simulink model "test_mdl_NI"  (R2018a)
settings: Solver=VariableStepAuto  StartTime=0.0  StopTime=10.0  RelTol=1e-3
(part 15 of 24)

== system test_mdl_NI/To_NI_HIL/Soft_ABS/WheelSpeed ==
  in : Inport
  WhlFl_W_Meas : Subsystem
  WhlFr_W_Meas : Subsystem
  WhlRl_W_Meas : Subsystem
  WhlRotatFl_No_Cnt : Subsystem
  WhlRotatFr_No_Cnt : Subsystem
  WhlRotatRl_No_Cnt : Subsystem
  WhlRotatRr_No_Cnt : Subsystem
  WhlRr_W_Meas : Subsystem
  bus_creator : BusCreator  Inputs=8
  bus_selector : BusSelector  OutputSignals=WhlFl_W_Meas,WhlFr_W_Meas,WhlRl_W_Meas,WhlRr_W_Meas,WhlRotatFl_No_Cnt,WhlRotatFr_No_Cnt,WhlRotatRl_No_Cnt,WhlRotatRr_No_Cnt
  out_port : Outport
  wires:
  bus_creator/1 -> out_port/1  "WheelSpeed"
  WhlFl_W_Meas/1(out) -> bus_creator/1  "WhlFl_W_Meas"
  WhlFr_W_Meas/1(out) -> bus_creator/2  "WhlFr_W_Meas"
  WhlRl_W_Meas/1(out) -> bus_creator/3  "WhlRl_W_Meas"
  WhlRr_W_Meas/1(out) -> bus_creator/4  "WhlRr_W_Meas"
  WhlRotatFl_No_Cnt/1(out) -> bus_creator/5  "WhlRotatFl_No_Cnt"
  WhlRotatFr_No_Cnt/1(out) -> bus_creator/6  "WhlRotatFr_No_Cnt"
  WhlRotatRl_No_Cnt/1(out) -> bus_creator/7  "WhlRotatRl_No_Cnt"
  WhlRotatRr_No_Cnt/1(out) -> bus_creator/8  "WhlRotatRr_No_Cnt"
  bus_selector/1 -> WhlFl_W_Meas/1(in)  "<WhlFl_W_Meas>"
  bus_selector/2 -> WhlFr_W_Meas/1(in)  "<WhlFr_W_Meas>"
  bus_selector/3 -> WhlRl_W_Meas/1(in)  "<WhlRl_W_Meas>"
  bus_selector/4 -> WhlRr_W_Meas/1(in)  "<WhlRr_W_Meas>"
  bus_selector/5 -> WhlRotatFl_No_Cnt/1(in)  "<WhlRotatFl_No_Cnt>"
  bus_selector/6 -> WhlRotatFr_No_Cnt/1(in)  "<WhlRotatFr_No_Cnt>"
  bus_selector/7 -> WhlRotatRl_No_Cnt/1(in)  "<WhlRotatRl_No_Cnt>"
  bus_selector/8 -> WhlRotatRr_No_Cnt/1(in)  "<WhlRotatRr_No_Cnt>"
  in/1 -> bus_selector/1

== system test_mdl_NI/To_NI_HIL/Soft_ABS/Yaw_Data ==
  in : Inport
  VehYaw_W_Actl : Subsystem
  bus_creator : BusCreator  Inputs=1
  bus_selector : BusSelector  OutputSignals=VehYaw_W_Actl
  out_port : Outport
  wires:
  bus_creator/1 -> out_port/1  "Yaw_Data"
  VehYaw_W_Actl/1(out) -> bus_creator/1  "VehYaw_W_Actl"
  bus_selector/1 -> VehYaw_W_Actl/1(in)  "<VehYaw_W_Actl>"
  in/1 -> bus_selector/1

== system test_mdl_NI/To_NI_HIL/Soft_BCM/BodyInfo_3 ==
  in : Inport
  Ignition_Status : Subsystem
  bus_creator : BusCreator  Inputs=1
  bus_selector : BusSelector  OutputSignals=Ignition_Status
  out_port : Outport
  wires:
  bus_creator/1 -> out_port/1  "BodyInfo_3"
  Ignition_Status/1(out) -> bus_creator/1  "Ignition_Status"
  bus_selector/1 -> Ignition_Status/1(in)  "<Ignition_Status>"
  in/1 -> bus_selector/1

== system test_mdl_NI/To_NI_HIL/Soft_BCM/Cluster_Info1 ==
  in : Inport
  OdometerMasterValue : Subsystem
  OdometerMasterValue_UB : Subsystem
  bus_creator : BusCreator  Inputs=2
  bus_selector : BusSelector  OutputSignals=OdometerMasterValue,OdometerMasterValue_UB
  out_port : Outport
  wires:
  bus_creator/1 -> out_port/1  "Cluster_Info1"
  OdometerMasterValue/1(out) -> bus_creator/1  "OdometerMasterValue"
  OdometerMasterValue_UB/1(out) -> bus_creator/2  "OdometerMasterValue_UB"
  bus_selector/1 -> OdometerMasterValue/1(in)  "<OdometerMasterValue>"
  bus_selector/2 -> OdometerMasterValue_UB/1(in)  "<OdometerMasterValue_UB>"
  in/1 -> bus_selector/1

== system test_mdl_NI/To_NI_HIL/Soft_BCM/GGCC_Config_Mgmt_ID ==
  in : Inport
  Byte_0 : Subsystem
  Byte_1 : Subsystem
  Byte_2 : Subsystem
  Byte_3 : Subsystem
  Byte_4 : Subsystem
  Byte_5 : Subsystem
  Byte_6 : Subsystem
  Byte_7 : Subsystem
  bus_creator : BusCreator  Inputs=8
  bus_selector : BusSelector  OutputSignals=Byte_0,Byte_1,Byte_2,Byte_3,Byte_4,Byte_5,Byte_6,Byte_7
  out_port : Outport
  wires:
  bus_creator/1 -> out_port/1  "GGCC_Config_Mgmt_ID"
  Byte_0/1(out) -> bus_creator/1  "Byte_0"
  Byte_1/1(out) -> bus_creator/2  "Byte_1"
  Byte_2/1(out) -> bus_creator/3  "Byte_2"
  Byte_3/1(out) -> bus_creator/4  "Byte_3"
  Byte_4/1(out) -> bus_creator/5  "Byte_4"
  Byte_5/1(out) -> bus_creator/6  "Byte_5"
  Byte_6/1(out) -> bus_creator/7  "Byte_6"
  Byte_7/1(out) -> bus_creator/8  "Byte_7"
  bus_selector/1 -> Byte_0/1(in)  "<Byte_0>"
  bus_selector/2 -> Byte_1/1(in)  "<Byte_1>"
  bus_selector/3 -> Byte_2/1(in)  "<Byte_2>"
  bus_selector/4 -> Byte_3/1(in)  "<Byte_3>"
  bus_selector/5 -> Byte_4/1(in)  "<Byte_4>"
  bus_selector/6 -> Byte_5/1(in)  "<Byte_5>"
  bus_selector/7 -> Byte_6/1(in)  "<Byte_6>"
  bus_selector/8 -> Byte_7/1(in)  "<Byte_7>"
  in/1 -> bus_selector/1

== system test_mdl_NI/To_NI_HIL/Soft_BCM/Personality_BCM2_Data ==
  in : Inport
  RecallEvent_No_Cnt : Subsystem
  bus_creator : BusCreator  Inputs=1
  bus_selector : BusSelector  OutputSignals=RecallEvent_No_Cnt
  out_port : Outport
  wires:
  bus_creator/1 -> out_port/1  "Personality_BCM2_Data"
  RecallEvent_No_Cnt/1(out) -> bus_creator/1  "RecallEvent_No_Cnt"
  bus_selector/1 -> RecallEvent_No_Cnt/1(in)  "<RecallEvent_No_Cnt>"
  in/1 -> bus_selector/1

== system test_mdl_NI/To_NI_HIL/Soft_BCM/signal1 ==
  in : Inport
  out : Outport
  wires:
  in/1 -> out/1

== system test_mdl_NI/To_NI_HIL/Soft_BCM/signal5 ==
  in : Inport
  out : Outport
  wires:
  in/1 -> out/1

== system test_mdl_NI/To_NI_HIL/Soft_BCM/signal6 ==
  in : Inport
  out : Outport
  wires:
  in/1 -> out/1

== system test_mdl_NI/To_NI_HIL/Soft_ECM/EngBrakeData ==
  in : Inport
  ACCStopMde_D_Rq : Subsystem
  Cc_Stat_D_Actl : Subsystem
  CmbbEngTqMn_B_Rq : Subsystem
  PrplTqMnSat_B_Actl : Subsystem
  bus_creator : BusCreator  Inputs=4
  bus_selector : BusSelector  OutputSignals=CmbbEngTqMn_B_Rq,ACCStopMde_D_Rq,PrplTqMnSat_B_Actl,Cc_Stat_D_Actl
  out_port : Outport
  wires:
  bus_creator/1 -> out_port/1  "EngBrakeData"
  CmbbEngTqMn_B_Rq/1(out) -> bus_creator/1  "CmbbEngTqMn_B_Rq"
  ACCStopMde_D_Rq/1(out) -> bus_creator/2  "ACCStopMde_D_Rq"
  PrplTqMnSat_B_Actl/1(out) -> bus_creator/3  "PrplTqMnSat_B_Actl"
  Cc_Stat_D_Actl/1(out) -> bus_creator/4  "Cc_Stat_D_Actl"
  bus_selector/1 -> CmbbEngTqMn_B_Rq/1(in)  "<CmbbEngTqMn_B_Rq>"
  bus_selector/2 -> ACCStopMde_D_Rq/1(in)  "<ACCStopMde_D_Rq>"
  bus_selector/3 -> PrplTqMnSat_B_Actl/1(in)  "<PrplTqMnSat_B_Actl>"
  bus_selector/4 -> Cc_Stat_D_Actl/1(in)  "<Cc_Stat_D_Actl>"
  in/1 -> bus_selector/1

== system test_mdl_NI/To_NI_HIL/Soft_ECM/EngVehicleSpThrottle ==
  in : Inport
  EngAout_N_Actl : Subsystem
  bus_creator : BusCreator  Inputs=1
  bus_selector : BusSelector  OutputSignals=EngAout_N_Actl
  out_port : Outport
  wires:
  bus_creator/1 -> out_port/1  "EngVehicleSpThrottle"
  EngAout_N_Actl/1(out) -> bus_creator/1  "EngAout_N_Actl"
  bus_selector/1 -> EngAout_N_Actl/1(in)  "<EngAout_N_Actl>"
  in/1 -> bus_selector/1

== system test_mdl_NI/To_NI_HIL/Soft_ECM/EngVehicleSpThrottle2 ==
  in : Inport
  Veh_V_ActlEng : Subsystem
  bus_creator : BusCreator  Inputs=1
  bus_selector : BusSelector  OutputSignals=Veh_V_ActlEng
  out_port : Outport
  wires:
  bus_creator/1 -> out_port/1  "EngVehicleSpThrottle2"
  Veh_V_ActlEng/1(out) -> bus_creator/1  "Veh_V_ActlEng"
  bus_selector/1 -> Veh_V_ActlEng/1(in)  "<Veh_V_ActlEng>"
  in/1 -> bus_selector/1

== system test_mdl_NI/To_NI_HIL/Soft_MRR/MRR_Detection ==
  in : Inport
  MRR_Detection_001 : Subsystem
  MRR_Detection_002 : Subsystem
  MRR_Detection_003 : Subsystem
  bus_creator : BusCreator  Inputs=3
  bus_selector : BusSelector  OutputSignals=MRR_Detection_001,MRR_Detection_002,MRR_Detection_003
  out_port : Outport
  wires:
  bus_creator/1 -> out_port/1  "MRR_Detection"
  MRR_Detection_001/1(out_port) -> bus_creator/1  "MRR_Detection_001"
  MRR_Detection_002/1(out_port) -> bus_creator/2  "MRR_Detection_002"
  MRR_Detection_003/1(out_port) -> bus_creator/3  "MRR_Detection_003"
  bus_selector/1 -> MRR_Detection_001/1(in)  "<MRR_Detection_001>"
  bus_selector/2 -> MRR_Detection_002/1(in)  "<MRR_Detection_002>"
  bus_selector/3 -> MRR_Detection_003/1(in)  "<MRR_Detection_003>"
  in/1 -> bus_selector/1

== system test_mdl_NI/To_NI_HIL/Soft_MRR/NumOfDetections ==
  in : Inport
  out : Outport
  wires:
  in/1 -> out/1

== system test_mdl_NI/To_NI_HIL/Soft_PCM/EngBrakeData ==
  in : Inport
  BpedDrvAppl_D_Actl : Subsystem
  BrkOnOffSwtch_D_Actl : Subsystem
  bus_creator : BusCreator  Inputs=2
  bus_selector : BusSelector  OutputSignals=BrkOnOffSwtch_D_Actl,BpedDrvAppl_D_Actl
  out_port : Outport
  wires:
  bus_creator/1 -> out_port/1  "EngBrakeData"
  BrkOnOffSwtch_D_Actl/1(out) -> bus_creator/1  "BrkOnOffSwtch_D_Actl"
  BpedDrvAppl_D_Actl/1(out) -> bus_creator/2  "BpedDrvAppl_D_Actl"
  bus_selector/1 -> BrkOnOffSwtch_D_Actl/1(in)  "<BrkOnOffSwtch_D_Actl>"
  bus_selector/2 -> BpedDrvAppl_D_Actl/1(in)  "<BpedDrvAppl_D_Actl>"
  in/1 -> bus_selector/1

== system test_mdl_NI/To_NI_HIL/Soft_PCM/EngVehicleSpThottle2 ==
  in : Inport
  GearRvrse_D_Actl : Subsystem
  Veh_V_ActlEng : Subsystem
  Veh_V_RqCcSet : Subsystem
  bus_creator : BusCreator  Inputs=3
  bus_selector : BusSelector  OutputSignals=Veh_V_ActlEng,GearRvrse_D_Actl,Veh_V_RqCcSet
  out_port : Outport
  wires:
  bus_creator/1 -> out_port/1  "EngVehicleSpThottle2"
  Veh_V_ActlEng/1(out) -> bus_creator/1  "Veh_V_ActlEng"
  GearRvrse_D_Actl/1(out) -> bus_creator/2  "GearRvrse_D_Actl"
  Veh_V_RqCcSet/1(out) -> bus_creator/3  "Veh_V_RqCcSet"
  bus_selector/1 -> Veh_V_ActlEng/1(in)  "<Veh_V_ActlEng>"
  bus_selector/2 -> GearRvrse_D_Actl/1(in)  "<GearRvrse_D_Actl>"
  bus_selector/3 -> Veh_V_RqCcSet/1(in)  "<Veh_V_RqCcSet>"
  in/1 -> bus_selector/1

== system test_mdl_NI/To_NI_HIL/Soft_PCM/EngVehicleSpThrottle ==
  in : Inport
  ApedPosPcActl_No_Cs : Subsystem
  ApedPos_PcRate_ActlArb : Subsystem
  ApedPos_Pc_ActlArb : Subsystem
  ApedPos_Pc_ActlArb_No_Cnt : Subsystem
  EngAout_N_Actl : Subsystem
  bus_creator : BusCreator  Inputs=5
  bus_selector : BusSelector  OutputSignals=EngAout_N_Actl,ApedPos_Pc_ActlArb,ApedPos_PcRate_ActlArb,ApedPosPcActl_No_Cs,ApedPos_Pc_ActlArb_No_Cnt
  out_port : Outport
  wires:
  bus_creator/1 -> out_port/1  "EngVehicleSpThrottle"
  EngAout_N_Actl/1(out) -> bus_creator/1  "EngAout_N_Actl"
  ApedPos_Pc_ActlArb/1(out) -> bus_creator/2  "ApedPos_Pc_ActlArb"
  ApedPos_PcRate_ActlArb/1(out) -> bus_creator/3  "ApedPos_PcRate_ActlArb"
  ApedPosPcActl_No_Cs/1(out) -> bus_creator/4  "ApedPosPcActl_No_Cs"
  ApedPos_Pc_ActlArb_No_Cnt/1(out) -> bus_creator/5  "ApedPos_Pc_ActlArb_No_Cnt"
  bus_selector/1 -> EngAout_N_Actl/1(in)  "<EngAout_N_Actl>"
  bus_selector/2 -> ApedPos_Pc_ActlArb/1(in)  "<ApedPos_Pc_ActlArb>"
  bus_selector/3 -> ApedPos_PcRate_ActlArb/1(in)  "<ApedPos_PcRate_ActlArb>"
  bus_selector/4 -> ApedPosPcActl_No_Cs/1(in)  "<ApedPosPcActl_No_Cs>"
  bus_selector/5 -> ApedPos_Pc_ActlArb_No_Cnt/1(in)  "<ApedPos_Pc_ActlArb_No_Cnt>"
  in/1 -> bus_selector/1

== system test_mdl_NI/To_NI_HIL/Soft_PCM/EngineClimateData ==
  in : Inport
  AirAmb_Te_Actl : Subsystem
  AirAmb_Te_ActlFilt : Subsystem
  EngAout_Aa_Actl : Subsystem
  bus_creator : BusCreator  Inputs=3
  bus_selector : BusSelector  OutputSignals=EngAout_Aa_Actl,AirAmb_Te_Actl,AirAmb_Te_ActlFilt
  out_port : Outport
  wires:
  bus_creator/1 -> out_port/1  "EngineClimateData"
  EngAout_Aa_Actl/1(out) -> bus_creator/1  "EngAout_Aa_Actl"
  AirAmb_Te_Actl/1(out) -> bus_creator/2  "AirAmb_Te_Actl"
  AirAmb_Te_ActlFilt/1(out) -> bus_creator/3  "AirAmb_Te_ActlFilt"
  bus_selector/1 -> EngAout_Aa_Actl/1(in)  "<EngAout_Aa_Actl>"
  bus_selector/2 -> AirAmb_Te_Actl/1(in)  "<AirAmb_Te_Actl>"
  bus_selector/3 -> AirAmb_Te_ActlFilt/1(in)  "<AirAmb_Te_ActlFilt>"
  in/1 -> bus_selector/1

== system test_mdl_NI/To_NI_HIL/Soft_PCM/EngineClutchData ==
  in : Inport
  CluPdlPosPcMeas_D_Qf : Subsystem
  CluPdlPos_Pc_Meas : Subsystem
  CluPdl_PcRate_Actl : Subsystem
  bus_creator : BusCreator  Inputs=3
  bus_selector : BusSelector  OutputSignals=CluPdl_PcRate_Actl,CluPdlPos_Pc_Meas,CluPdlPosPcMeas_D_Qf
  out_port : Outport
  wires:
  bus_creator/1 -> out_port/1  "EngineClutchData"
  CluPdl_PcRate_Actl/1(out) -> bus_creator/1  "CluPdl_PcRate_Actl"
  CluPdlPos_Pc_Meas/1(out) -> bus_creator/2  "CluPdlPos_Pc_Meas"
  CluPdlPosPcMeas_D_Qf/1(out) -> bus_creator/3  "CluPdlPosPcMeas_D_Qf"
  bus_selector/1 -> CluPdl_PcRate_Actl/1(in)  "<CluPdl_PcRate_Actl>"
  bus_selector/2 -> CluPdlPos_Pc_Meas/1(in)  "<CluPdlPos_Pc_Meas>"
  bus_selector/3 -> CluPdlPosPcMeas_D_Qf/1(in)  "<CluPdlPosPcMeas_D_Qf>"
  in/1 -> bus_selector/1

== system test_mdl_NI/To_NI_HIL/Soft_PCM/EngineData_7 ==
  in : Inport
  FuelFlw_Vl_Dsply : Subsystem
  OdoCount : Subsystem
  bus_creator : BusCreator  Inputs=2
  bus_selector : BusSelector  OutputSignals=OdoCount,FuelFlw_Vl_Dsply
  out_port : Outport
  wires:
  bus_creator/1 -> out_port/1  "EngineData_7"
  OdoCount/1(out) -> bus_creator/1  "OdoCount"
  FuelFlw_Vl_Dsply/1(out) -> bus_creator/2  "FuelFlw_Vl_Dsply"
  bus_selector/1 -> OdoCount/1(in)  "<OdoCount>"
  bus_selector/2 -> FuelFlw_Vl_Dsply/1(in)  "<FuelFlw_Vl_Dsply>"
  in/1 -> bus_selector/1

== system test_mdl_NI/To_NI_HIL/Soft_PCM/PowertrainData_10 ==
  in : Inport
  GearLvr_D_ActlDrv : Subsystem
  GearPos_No_Cnt : Subsystem
  GearPos_No_Cs : Subsystem
  bus_creator : BusCreator  Inputs=3
  bus_selector : BusSelector  OutputSignals=GearPos_No_Cs,GearPos_No_Cnt,GearLvr_D_ActlDrv
  out_port : Outport
  wires:
  bus_creator/1 -> out_port/1  "PowertrainData_10"
  GearPos_No_Cs/1(out) -> bus_creator/1  "GearPos_No_Cs"
  GearPos_No_Cnt/1(out) -> bus_creator/2  "GearPos_No_Cnt"
  GearLvr_D_ActlDrv/1(out) -> bus_creator/3  "GearLvr_D_ActlDrv"
  bus_selector/1 -> GearPos_No_Cs/1(in)  "<GearPos_No_Cs>"
  bus_selector/2 -> GearPos_No_Cnt/1(in)  "<GearPos_No_Cnt>"
  bus_selector/3 -> GearLvr_D_ActlDrv/1(in)  "<GearLvr_D_ActlDrv>"
  in/1 -> bus_selector/1

== system test_mdl_NI/To_NI_HIL/Soft_PCM/TorqueDataEngFlags ==
  in : Inport
  PrplWhlTotTqRq_No_Cs : Subsystem
  PrplWhlTot_Tq_Rq : Subsystem
  PrplWhlTot_Tq_Rq_No_Cnt : Subsystem
  bus_creator : BusCreator  Inputs=3
  bus_selector : BusSelector  OutputSignals=PrplWhlTot_Tq_Rq,PrplWhlTotTqRq_No_Cs,PrplWhlTot_Tq_Rq_No_Cnt
  out_port : Outport
  wires:
  bus_creator/1 -> out_port/1  "TorqueDataEngFlags"
  PrplWhlTot_Tq_Rq/1(out) -> bus_creator/1  "PrplWhlTot_Tq_Rq"
  PrplWhlTotTqRq_No_Cs/1(out) -> bus_creator/2  "PrplWhlTotTqRq_No_Cs"
  PrplWhlTot_Tq_Rq_No_Cnt/1(out) -> bus_creator/3  "PrplWhlTot_Tq_Rq_No_Cnt"
  bus_selector/1 -> PrplWhlTot_Tq_Rq/1(in)  "<PrplWhlTot_Tq_Rq>"
  bus_selector/2 -> PrplWhlTotTqRq_No_Cs/1(in)  "<PrplWhlTotTqRq_No_Cs>"
  bus_selector/3 -> PrplWhlTot_Tq_Rq_No_Cnt/1(in)  "<PrplWhlTot_Tq_Rq_No_Cnt>"
  in/1 -> bus_selector/1

== system test_mdl_NI/To_NI_HIL/Soft_PCM/VehicleOperatingModes ==
  in : Inport
  ElPw_D_Stat : Subsystem
  ElPw_D_StatStrtStop : Subsystem
  Eng_D_Stat : Subsystem
  PrplWhlTot2_Tq_Rq : Subsystem
  PwPckTq_D_Stat : Subsystem
  bus_creator : BusCreator  Inputs=5
  bus_selector : BusSelector  OutputSignals=Eng_D_Stat,PwPckTq_D_Stat,PrplWhlTot2_Tq_Rq,ElPw_D_StatStrtStop,ElPw_D_Stat
  out_port : Outport
  wires:
  bus_creator/1 -> out_port/1  "VehicleOperatingModes"
  Eng_D_Stat/1(out) -> bus_creator/1  "Eng_D_Stat"
  PwPckTq_D_Stat/1(out) -> bus_creator/2  "PwPckTq_D_Stat"
  PrplWhlTot2_Tq_Rq/1(out) -> bus_creator/3  "PrplWhlTot2_Tq_Rq"
  ElPw_D_StatStrtStop/1(out) -> bus_creator/4  "ElPw_D_StatStrtStop"
  ElPw_D_Stat/1(out) -> bus_creator/5  "ElPw_D_Stat"
  bus_selector/1 -> Eng_D_Stat/1(in)  "<Eng_D_Stat>"
  bus_selector/2 -> PwPckTq_D_Stat/1(in)  "<PwPckTq_D_Stat>"
  bus_selector/3 -> PrplWhlTot2_Tq_Rq/1(in)  "<PrplWhlTot2_Tq_Rq>"
  bus_selector/4 -> ElPw_D_StatStrtStop/1(in)  "<ElPw_D_StatStrtStop>"
  bus_selector/5 -> ElPw_D_Stat/1(in)  "<ElPw_D_Stat>"
  in/1 -> bus_selector/1

== system test_mdl_NI/To_NI_HIL/Soft_PSCM/Angle_SteeringWheel ==
  in : Inport
  out : Outport
  wires:
  in/1 -> out/1

== system test_mdl_NI/To_NI_HIL/Soft_PSCM/StePinCompAnEst_D_Qf ==
  in : Inport
  out : Outport
  wires:
  in/1 -> out/1

== system test_mdl_NI/To_NI_HIL/Soft_PSCM/StePinRelInit_An_Sns ==
  in : Inport
  out : Outport
  wires:
  in/1 -> out/1

== system test_mdl_NI/To_NI_HIL/Soft_PSCM/StePw_B_Rq ==
  in : Inport
  out : Outport
  wires:
  in/1 -> out/1

== system test_mdl_NI/To_NI_HIL/Soft_PSCM/SteWhlAngCounter ==
  in : Inport
  out : Outport
  wires:
  in/1 -> out/1

== system test_mdl_NI/To_NI_HIL/Soft_PSCM/WhlAngleCs ==
  in : Inport
  out : Outport
  wires:
  in/1 -> out/1

== system test_mdl_NI/To_NI_HIL/Soft_RCM/Accel_Data ==
  in : Inport
  VehLat2_A_Actl : Subsystem
  VehLatAActl_D_Qf : Subsystem
  VehLatLongVert_No_Cnt : Subsystem
  VehLatLongVert_No_Cs : Subsystem
  VehLong2_A_Actl : Subsystem
  VehLongAActl_D_Qf : Subsystem
  VehVert2_A_Actl : Subsystem
  VehVertAActl_D_Qf : Subsystem
  bus_creator : BusCreator  Inputs=8
  bus_selector : BusSelector  OutputSignals=VehLat2_A_Actl,VehLong2_A_Actl,VehVert2_A_Actl,VehLatLongVert_No_Cnt,VehLatLongVert_No_Cs,VehLatAActl_D_Qf,VehLongAActl_D_Qf,VehVertAActl_D_Qf
  out_port : Outport
  wires:
  bus_creator/1 -> out_port/1  "Accel_Data"
  VehLat2_A_Actl/1(out) -> bus_creator/1  "VehLat2_A_Actl"
  VehLong2_A_Actl/1(out) -> bus_creator/2  "VehLong2_A_Actl"
  VehVert2_A_Actl/1(out) -> bus_creator/3  "VehVert2_A_Actl"
  VehLatLongVert_No_Cnt/1(out) -> bus_creator/4  "VehLatLongVert_No_Cnt"
  VehLatLongVert_No_Cs/1(out) -> bus_creator/5  "VehLatLongVert_No_Cs"
  VehLatAActl_D_Qf/1(out) -> bus_creator/6  "VehLatAActl_D_Qf"
  VehLongAActl_D_Qf/1(out) -> bus_creator/7  "VehLongAActl_D_Qf"
  VehVertAActl_D_Qf/1(out) -> bus_creator/8  "VehVertAActl_D_Qf"
  bus_selector/1 -> VehLat2_A_Actl/1(in)  "<VehLat2_A_Actl>"
  bus_selector/2 -> VehLong2_A_Actl/1(in)  "<VehLong2_A_Actl>"
  bus_selector/3 -> VehVert2_A_Actl/1(in)  "<VehVert2_A_Actl>"
  bus_selector/4 -> VehLatLongVert_No_Cnt/1(in)  "<VehLatLongVert_No_Cnt>"
  bus_selector/5 -> VehLatLongVert_No_Cs/1(in)  "<VehLatLongVert_No_Cs>"
  bus_selector/6 -> VehLatAActl_D_Qf/1(in)  "<VehLatAActl_D_Qf>"
  bus_selector/7 -> VehLongAActl_D_Qf/1(in)  "<VehLongAActl_D_Qf>"
  bus_selector/8 -> VehVertAActl_D_Qf/1(in)  "<VehVertAActl_D_Qf>"
  in/1 -> bus_selector/1

== system test_mdl_NI/To_NI_HIL/Soft_RCM/RCMStatusMessage2 ==
  in : Inport
  FirstRowBuckleDriver : Subsystem
  RstrnImpactEvntStatus : Subsystem
  bus_creator : BusCreator  Inputs=2
  bus_selector : BusSelector  OutputSignals=RstrnImpactEvntStatus,FirstRowBuckleDriver
  out_port : Outport
  wires:
  bus_creator/1 -> out_port/1  "RCMStatusMessage2"
  RstrnImpactEvntStatus/1(out) -> bus_creator/1  "RstrnImpactEvntStatus"
  FirstRowBuckleDriver/1(out) -> bus_creator/2  "FirstRowBuckleDriver"
  bus_selector/1 -> RstrnImpactEvntStatus/1(in)  "<RstrnImpactEvntStatus>"
  bus_selector/2 -> FirstRowBuckleDriver/1(in)  "<FirstRowBuckleDriver>"
  in/1 -> bus_selector/1

== system test_mdl_NI/To_NI_HIL/Soft_RCM/Yaw_Data ==
  in : Inport
  VehRolWActl_D_Qf : Subsystem
  VehRol_W_Actl : Subsystem
  VehRollYawW_No_Cs : Subsystem
  VehRollYaw_No_Cnt : Subsystem
  VehYawWActl_D_Qf : Subsystem
  VehYaw_W_Actl : Subsystem
  bus_creator : BusCreator  Inputs=6
  bus_selector : BusSelector  OutputSignals=VehRol_W_Actl,VehYaw_W_Actl,VehRollYaw_No_Cnt,VehRollYawW_No_Cs,VehRolWActl_D_Qf,VehYawWActl_D_Qf
  out_port : Outport
  wires:
  bus_creator/1 -> out_port/1  "Yaw_Data"
  VehRol_W_Actl/1(out) -> bus_creator/1  "VehRol_W_Actl"
  VehYaw_W_Actl/1(out) -> bus_creator/2  "VehYaw_W_Actl"
  VehRollYaw_No_Cnt/1(out) -> bus_creator/3  "VehRollYaw_No_Cnt"
  VehRollYawW_No_Cs/1(out) -> bus_creator/4  "VehRollYawW_No_Cs"
  VehRolWActl_D_Qf/1(out) -> bus_creator/5  "VehRolWActl_D_Qf"
  VehYawWActl_D_Qf/1(out) -> bus_creator/6  "VehYawWActl_D_Qf"
  bus_selector/1 -> VehRol_W_Actl/1(in)  "<VehRol_W_Actl>"
  bus_selector/2 -> VehYaw_W_Actl/1(in)  "<VehYaw_W_Actl>"
  bus_selector/3 -> VehRollYaw_No_Cnt/1(in)  "<VehRollYaw_No_Cnt>"
  bus_selector/4 -> VehRollYawW_No_Cs/1(in)  "<VehRollYawW_No_Cs>"
  bus_selector/5 -> VehRolWActl_D_Qf/1(in)  "<VehRolWActl_D_Qf>"
  bus_selector/6 -> VehYawWActl_D_Qf/1(in)  "<VehYawWActl_D_Qf>"
  in/1 -> bus_selector/1

== system test_mdl_NI/To_NI_HIL/Soft_SCCM/Steering_Data ==
  in : Inport
  AccButtnGapDecPress : Subsystem
  AccButtnGapIncPress : Subsystem
  AhbStat_B_Dsply : Subsystem
  AslButtnOnOffCnclPress : Subsystem
  AslButtnOnOffPress : Subsystem
  CcAslButtnCnclPress : Subsystem
  CcAslButtnCnclResPress : Subsystem
  CcAslButtnOnPress : Subsystem
  CcAslButtnResDecPress : Subsystem
  CcAslButtnResIncPress : Subsystem
  CcAslButtnSetDecPress : Subsystem
  CcAslButtnSetIncPress : Subsystem
  CcAslButtnSetPress : Subsystem
  CcAsllButtnResPress : Subsystem
  CcButtnOffPress : Subsystem
  CcButtnOnOffCnclPress : Subsystem
  CcButtnOnOffPress : Subsystem
  CcButtnOnPress : Subsystem
  HeadLghtHiCtrl_D_RqAhb : Subsystem
  HeadLghtHiOn_B_StatAhb : Subsystem
  bus_creator : BusCreator  Inputs=20
  bus_selector : BusSelector  OutputSignals=AhbStat_B_Dsply,HeadLghtHiCtrl_D_RqAhb,HeadLghtHiOn_B_StatAhb,CcButtnOnPress,CcButtnOffPress,CcAslButtnCnclPress,CcAsllButtnResPress,CcAslButtnResIncPress,CcAslButtnSetIncPress,CcAslButtnSetDecPress,CcAslButtnSetPress,AccButtnGapIncPress,AccButtnGapDecPress,AslButtnOnOffPress,AslButtnOnOffCnclPress,CcButtnOnOffPress,CcButtnOnOffCnclPress,CcAslButtnResDecPress,CcAslButtnOnPress,CcAslButtnCnclResPress
  out_port : Outport
  wires:
  bus_creator/1 -> out_port/1  "Steering_Data"
  AhbStat_B_Dsply/1(out) -> bus_creator/1  "AhbStat_B_Dsply"
  HeadLghtHiCtrl_D_RqAhb/1(out) -> bus_creator/2  "HeadLghtHiCtrl_D_RqAhb"
  HeadLghtHiOn_B_StatAhb/1(out) -> bus_creator/3  "HeadLghtHiOn_B_StatAhb"
  CcButtnOnPress/1(out) -> bus_creator/4  "CcButtnOnPress"
  CcButtnOffPress/1(out) -> bus_creator/5  "CcButtnOffPress"
  CcAslButtnCnclPress/1(out) -> bus_creator/6  "CcAslButtnCnclPress"
  CcAsllButtnResPress/1(out) -> bus_creator/7  "CcAsllButtnResPress"
  CcAslButtnResIncPress/1(out) -> bus_creator/8  "CcAslButtnResIncPress"
  CcAslButtnSetIncPress/1(out) -> bus_creator/9  "CcAslButtnSetIncPress"
  CcAslButtnSetDecPress/1(out) -> bus_creator/10  "CcAslButtnSetDecPress"
  CcAslButtnSetPress/1(out) -> bus_creator/11  "CcAslButtnSetPress"
  AccButtnGapIncPress/1(out) -> bus_creator/12  "AccButtnGapIncPress"
  AccButtnGapDecPress/1(out) -> bus_creator/13  "AccButtnGapDecPress"
  AslButtnOnOffPress/1(out) -> bus_creator/14  "AslButtnOnOffPress"
  AslButtnOnOffCnclPress/1(out) -> bus_creator/15  "AslButtnOnOffCnclPress"
  CcButtnOnOffPress/1(out) -> bus_creator/16  "CcButtnOnOffPress"
  CcButtnOnOffCnclPress/1(out) -> bus_creator/17  "CcButtnOnOffCnclPress"
  CcAslButtnResDecPress/1(out) -> bus_creator/18  "CcAslButtnResDecPress"
  CcAslButtnOnPress/1(out) -> bus_creator/19  "CcAslButtnOnPress"
  CcAslButtnCnclResPress/1(out) -> bus_creator/20  "CcAslButtnCnclResPress"
  bus_selector/1 -> AhbStat_B_Dsply/1(in)  "<AhbStat_B_Dsply>"
  bus_selector/2 -> HeadLghtHiCtrl_D_RqAhb/1(in)  "<HeadLghtHiCtrl_D_RqAhb>"
  bus_selector/3 -> HeadLghtHiOn_B_StatAhb/1(in)  "<HeadLghtHiOn_B_StatAhb>"
  bus_selector/4 -> CcButtnOnPress/1(in)  "<CcButtnOnPress>"
  bus_selector/5 -> CcButtnOffPress/1(in)  "<CcButtnOffPress>"
  bus_selector/6 -> CcAslButtnCnclPress/1(in)  "<CcAslButtnCnclPress>"
  bus_selector/7 -> CcAsllButtnResPress/1(in)  "<CcAsllButtnResPress>"
  bus_selector/8 -> CcAslButtnResIncPress/1(in)  "<CcAslButtnResIncPress>"
  bus_selector/9 -> CcAslButtnSetIncPress/1(in)  "<CcAslButtnSetIncPress>"
  bus_selector/10 -> CcAslButtnSetDecPress/1(in)  "<CcAslButtnSetDecPress>"
  bus_selector/11 -> CcAslButtnSetPress/1(in)  "<CcAslButtnSetPress>"
  bus_selector/12 -> AccButtnGapIncPress/1(in)  "<AccButtnGapIncPress>"
  bus_selector/13 -> AccButtnGapDecPress/1(in)  "<AccButtnGapDecPress>"
  bus_selector/14 -> AslButtnOnOffPress/1(in)  "<AslButtnOnOffPress>"
  bus_selector/15 -> AslButtnOnOffCnclPress/1(in)  "<AslButtnOnOffCnclPress>"
  bus_selector/16 -> CcButtnOnOffPress/1(in)  "<CcButtnOnOffPress>"
  bus_selector/17 -> CcButtnOnOffCnclPress/1(in)  "<CcButtnOnOffCnclPress>"
  bus_selector/18 -> CcAslButtnResDecPress/1(in)  "<CcAslButtnResDecPress>"
  bus_selector/19 -> CcAslButtnOnPress/1(in)  "<CcAslButtnOnPress>"
  bus_selector/20 -> CcAslButtnCnclResPress/1(in)  "<CcAslButtnCnclResPress>"
  in/1 -> bus_selector/1

== system test_mdl_NI/To_NI_HIL/Soft_SCCM/Steering_Wheel_Data2 ==
  in : Inport
  SteWhlSwtchBack_B_Stat : Subsystem
  SteWhlSwtchDown_B_Stat : Subsystem
  SteWhlSwtchLeft_B_Stat : Subsystem
  SteWhlSwtchMenu_B_Stat : Subsystem
  SteWhlSwtchOk_B_Stat : Subsystem
  SteWhlSwtchRght_B_Stat : Subsystem
  SteWhlSwtchUp_B_Stat : Subsystem
  bus_creator : BusCreator  Inputs=7
  bus_selector : BusSelector  OutputSignals=SteWhlSwtchOk_B_Stat,SteWhlSwtchUp_B_Stat,SteWhlSwtchDown_B_Stat,SteWhlSwtchLeft_B_Stat,SteWhlSwtchRght_B_Stat,SteWhlSwtchMenu_B_Stat,SteWhlSwtchBack_B_Stat
  out_port : Outport
  wires:
  bus_creator/1 -> out_port/1  "Steering_Wheel_Data2"
  SteWhlSwtchOk_B_Stat/1(out) -> bus_creator/1  "SteWhlSwtchOk_B_Stat"
  SteWhlSwtchUp_B_Stat/1(out) -> bus_creator/2  "SteWhlSwtchUp_B_Stat"
  SteWhlSwtchDown_B_Stat/1(out) -> bus_creator/3  "SteWhlSwtchDown_B_Stat"
  SteWhlSwtchLeft_B_Stat/1(out) -> bus_creator/4  "SteWhlSwtchLeft_B_Stat"
  SteWhlSwtchRght_B_Stat/1(out) -> bus_creator/5  "SteWhlSwtchRght_B_Stat"
  SteWhlSwtchMenu_B_Stat/1(out) -> bus_creator/6  "SteWhlSwtchMenu_B_Stat"
  SteWhlSwtchBack_B_Stat/1(out) -> bus_creator/7  "SteWhlSwtchBack_B_Stat"
  bus_selector/1 -> SteWhlSwtchOk_B_Stat/1(in)  "<SteWhlSwtchOk_B_Stat>"
  bus_selector/2 -> SteWhlSwtchUp_B_Stat/1(in)  "<SteWhlSwtchUp_B_Stat>"
  bus_selector/3 -> SteWhlSwtchDown_B_Stat/1(in)  "<SteWhlSwtchDown_B_Stat>"
  bus_selector/4 -> SteWhlSwtchLeft_B_Stat/1(in)  "<SteWhlSwtchLeft_B_Stat>"
  bus_selector/5 -> SteWhlSwtchRght_B_Stat/1(in)  "<SteWhlSwtchRght_B_Stat>"
  bus_selector/6 -> SteWhlSwtchMenu_B_Stat/1(in)  "<SteWhlSwtchMenu_B_Stat>"
  bus_selector/7 -> SteWhlSwtchBack_B_Stat/1(in)  "<SteWhlSwtchBack_B_Stat>"
  in/1 -> bus_selector/1

== system test_mdl_NI/To_NI_HIL/Soft_TCM/TransGearData ==
  in : Inport
  GearLvrPos_D_Actl : Subsystem
  bus_creator : BusCreator  Inputs=1
  bus_selector : BusSelector  OutputSignals=GearLvrPos_D_Actl
  out_port : Outport
  wires:
  bus_creator/1 -> out_port/1  "TransGearData"
  GearLvrPos_D_Actl/1(out) -> bus_creator/1  "GearLvrPos_D_Actl"
  bus_selector/1 -> GearLvrPos_D_Actl/1(in)  "<GearLvrPos_D_Actl>"
  in/1 -> bus_selector/1

== system test_mdl_NI/CAN_Signal/ABS_ESC/ABS_AutoSar_NetworkMgt_0x596/ABS_AutoSarNMControl ==
  in : Inport
  out : Outport
  wires:
  in/1 -> out/1

== system test_mdl_NI/CAN_Signal/ABS_ESC/ABS_AutoSar_NetworkMgt_0x596/ABS_AutoSarNMNodeId ==
  in : Inport
  out : Outport
  wires:
  in/1 -> out/1

== system test_mdl_NI/CAN_Signal/ABS_ESC/ABS_AutoSar_NetworkMgt_0x596/ABS_AutoSarNMReserved1 ==
  in : Inport
  out : Outport
  wires:
  in/1 -> out/1

== system test_mdl_NI/CAN_Signal/ABS_ESC/ABS_AutoSar_NetworkMgt_0x596/ABS_AutoSarNMReserved2 ==
  in : Inport
  out : Outport
  wires:
  in/1 -> out/1

== system test_mdl_NI/CAN_Signal/ABS_ESC/ABS_AutoSar_NetworkMgt_0x596/ABS_AutoSarNMReserved3 ==
  in : Inport
  out : Outport
  wires:
  in/1 -> out/1

== system test_mdl_NI/CAN_Signal/ABS_ESC/ABS_AutoSar_NetworkMgt_0x596/ABS_AutoSarNMReserved4 ==
  in : Inport
  out : Outport
  wires:
  in/1 -> out/1

== system test_mdl_NI/CAN_Signal/ABS_ESC/ABS_AutoSar_NetworkMgt_0x596/ABS_GWNMProxy ==
  in : Inport
  out : Outport
  wires:
  in/1 -> out/1

== system test_mdl_NI/CAN_Signal/ABS_ESC/ABS_AutoSar_NetworkMgt_0x596/ABS_GWOnBoardTester ==
  in : Inport
  out : Outport
  wires:
  in/1 -> out/1

== system test_mdl_NI/CAN_Signal/ABS_ESC/ABS_BrkBst_Data_0x4B0/BrkAutoHold_D_Stat ==
  in : Inport
  out : Outport
  wires:
  in/1 -> out/1

== system test_mdl_NI/CAN_Signal/ABS_ESC/ABS_BrkBst_Data_0x4B0/BrkBstrVac_P_Actl ==
  in : Inport
  out : Outport
  wires:
  in/1 -> out/1

== system test_mdl_NI/CAN_Signal/ABS_ESC/ABS_BrkBst_Data_0x4B0/BrkTotTqRqDrv_No_Cnt ==
  in : Inport
  out : Outport
  wires:
  in/1 -> out/1

== system test_mdl_NI/CAN_Signal/ABS_ESC/ABS_BrkBst_Data_0x4B0/BrkTotTqRqDrv_No_Cs ==
  in : Inport
  out : Outport
  wires:
  in/1 -> out/1

== system test_mdl_NI/CAN_Signal/ABS_ESC/ABS_BrkBst_Data_0x4B0/BrkTot_Tq_RqDrv ==
  in : Inport
  out : Outport
  wires:
  in/1 -> out/1

== system test_mdl_NI/CAN_Signal/ABS_ESC/ABS_BrkBst_Data_0x4B0/HsaStat_D_Dsply ==
  in : Inport
  out : Outport
  wires:
  in/1 -> out/1

== system test_mdl_NI/CAN_Signal/ABS_ESC/ABS_BrkBst_Data_0x4B0/HsaTrnAout_Tq_Rq ==
  in : Inport
  out : Outport
  wires:
  in/1 -> out/1

== system test_mdl_NI/CAN_Signal/ABS_ESC/ABS_BrkBst_Data_0x4B0/YawStabilityIndex ==
  in : Inport
  out : Outport
  wires:
  in/1 -> out/1

== system test_mdl_NI/CAN_Signal/ABS_ESC/ABS_Rapid_Data_Response_1_0x6B0/UUDTABSResponse1 ==
  in : Inport
  out : Outport
  wires:
  in/1 -> out/1

== system test_mdl_NI/CAN_Signal/ABS_ESC/ABS_Rapid_Data_Response_2_0x6B1/UUDTABSResponse2 ==
  in : Inport
  out : Outport
  wires:
  in/1 -> out/1

== system test_mdl_NI/CAN_Signal/ABS_ESC/ActiveFronSteering_Req_0x88/SteWhlBrkAnRq_No_Cnt ==
  in : Inport
  out : Outport
  wires:
  in/1 -> out/1

== system test_mdl_NI/CAN_Signal/ABS_ESC/ActiveFronSteering_Req_0x88/SteWhlBrkAnRq_No_Cs ==
  in : Inport
  out : Outport
  wires:
  in/1 -> out/1

== system test_mdl_NI/CAN_Signal/ABS_ESC/ActiveFronSteering_Req_0x88/SteWhlBrkOffst_An_Rq ==
  in : Inport
  out : Outport
  wires:
  in/1 -> out/1

== system test_mdl_NI/CAN_Signal/ABS_ESC/BrakeSnData_3_0x77/VehLatComp_A_Actl ==
  in : Inport
  out : Outport
  wires:
  in/1 -> out/1

== system test_mdl_NI/CAN_Signal/ABS_ESC/BrakeSnData_3_0x77/VehLongComp_A_Actl ==
  in : Inport
  out : Outport
  wires:
  in/1 -> out/1

== system test_mdl_NI/CAN_Signal/ABS_ESC/BrakeSnData_3_0x77/VehOverGnd_V_Est ==
  in : Inport
  out : Outport
  wires:
  in/1 -> out/1

== system test_mdl_NI/CAN_Signal/ABS_ESC/BrakeSnData_3_0x77/VehTrvlDir_D_Stat ==
  in : Inport
  out : Outport
  wires:
  in/1 -> out/1

== system test_mdl_NI/CAN_Signal/ABS_ESC/BrakeSnData_3_0x77/VehYawComp_W_Actl ==
  in : Inport
  out : Outport
  wires:
  in/1 -> out/1

== system test_mdl_NI/CAN_Signal/ABS_ESC/BrakeSnData_4_0x7D/BrkTotTqRqArb_No_Cnt ==
  in : Inport
  out : Outport
  wires:
  in/1 -> out/1

== system test_mdl_NI/CAN_Signal/ABS_ESC/BrakeSnData_4_0x7D/BrkTotTqRqArb_No_Cs ==
  in : Inport
  out : Outport
  wires:
  in/1 -> out/1

== system test_mdl_NI/CAN_Signal/ABS_ESC/BrakeSnData_4_0x7D/BrkTot_Tq_Actl ==
  in : Inport
  out : Outport
  wires:
  in/1 -> out/1

== system test_mdl_NI/CAN_Signal/ABS_ESC/BrakeSnData_4_0x7D/BrkTot_Tq_RqArb ==
  in : Inport
  out : Outport
  wires:
  in/1 -> out/1

== system test_mdl_NI/CAN_Signal/ABS_ESC/BrakeSnData_4_0x7D/HsaStat_D_Actl ==
  in : Inport
  out : Outport
  wires:
  in/1 -> out/1

== system test_mdl_NI/CAN_Signal/ABS_ESC/BrakeSnData_4_0x7D/VehRolComp_W_Actl ==
  in : Inport
  out : Outport
  wires:
  in/1 -> out/1

== system test_mdl_NI/CAN_Signal/ABS_ESC/BrakeSnData_4_0x7D/VehVertComp_A_Actl ==
  in : Inport
  out : Outport
  wires:
  in/1 -> out/1

== system test_mdl_NI/CAN_Signal/ABS_ESC/BrakeSnData_5_0x76/AwdLck_Tq_RqMn ==
  in : Inport
  out : Outport
  wires:
  in/1 -> out/1

== system test_mdl_NI/CAN_Signal/ABS_ESC/BrakeSnData_5_0x76/AwdLck_Tq_RqMx ==
  in : Inport
  out : Outport
  wires:
  in/1 -> out/1

== system test_mdl_NI/CAN_Signal/ABS_ESC/BrakeSnData_5_0x76/BrkCtrFnd_B_Stat ==
  in : Inport
  out : Outport
  wires:
  in/1 -> out/1

== system test_mdl_NI/CAN_Signal/ABS_ESC/BrakeSnData_5_0x76/DrvSte_D_Stat ==
  in : Inport
  out : Outport
  wires:
  in/1 -> out/1

== system test_mdl_NI/CAN_Signal/ABS_ESC/BrakeSnData_5_0x76/DrvSte_Tq_Rq ==
  in : Inport
  out : Outport
  wires:
  in/1 -> out/1

== system test_mdl_NI/CAN_Signal/ABS_ESC/BrakeSnData_5_0x76/EmgcyBrkLamp_D_Rq ==
  in : Inport
  out : Outport
  wires:
  in/1 -> out/1

== system test_mdl_NI/CAN_Signal/ABS_ESC/BrakeSnData_5_0x76/SteWhlCompAnEst_D_Qf ==
  in : Inport
  out : Outport
  wires:
  in/1 -> out/1

== system test_mdl_NI/CAN_Signal/ABS_ESC/BrakeSnData_5_0x76/SteWhlComp_An_Est ==
  in : Inport
  out : Outport
  wires:
  in/1 -> out/1

== system test_mdl_NI/CAN_Signal/ABS_ESC/BrakeSnData_5_0x76/StopLamp_B_RqBrk ==
  in : Inport
  out : Outport
  wires:
  in/1 -> out/1

== system test_mdl_NI/CAN_Signal/ABS_ESC/BrakeSnData_6_0x414/StePinOffst_An_Est ==
  in : Inport
  out : Outport
  wires:
  in/1 -> out/1

== system test_mdl_NI/CAN_Signal/ABS_ESC/BrakeSnData_6_0x414/StePinOffst_D_Stat ==
  in : Inport
  out : Outport
  wires:
  in/1 -> out/1

== system test_mdl_NI/CAN_Signal/ABS_ESC/BrakeSnData_6_0x414/StePinOffst_No_Cnt ==
  in : Inport
  out : Outport
  wires:
  in/1 -> out/1

== system test_mdl_NI/CAN_Signal/ABS_ESC/BrakeSnData_6_0x414/StePinOffst_No_Cs ==
  in : Inport
  out : Outport
  wires:
  in/1 -> out/1

== system test_mdl_NI/CAN_Signal/ABS_ESC/BrakeSysFeatures_0x415/BrkFluidLvl_D_Stat ==
  in : Inport
  out : Outport
  wires:
  in/1 -> out/1

== system test_mdl_NI/CAN_Signal/ABS_ESC/BrakeSysFeatures_0x415/LsmcBrkDecel_D_Stat ==
  in : Inport
  out : Outport
  wires:
  in/1 -> out/1

== system test_mdl_NI/CAN_Signal/ABS_ESC/BrakeSysFeatures_0x415/VehStab_D_Stat ==
  in : Inport
  out : Outport
  wires:
  in/1 -> out/1

== system test_mdl_NI/CAN_Signal/ABS_ESC/BrakeSysFeatures_0x415/VehVActlBrk_D_Qf ==
  in : Inport
  out : Outport
  wires:
  in/1 -> out/1

== system test_mdl_NI/CAN_Signal/ABS_ESC/BrakeSysFeatures_0x415/VehVActlBrk_No_Cnt ==
  in : Inport
  out : Outport
  wires:
  in/1 -> out/1

== system test_mdl_NI/CAN_Signal/ABS_ESC/BrakeSysFeatures_0x415/VehVActlBrk_No_Cs ==
  in : Inport
  out : Outport
  wires:
  in/1 -> out/1

== system test_mdl_NI/CAN_Signal/ABS_ESC/BrakeSysFeatures_0x415/VehYawLin_W_Rq ==
  in : Inport
  out : Outport
  wires:
  in/1 -> out/1

== system test_mdl_NI/CAN_Signal/ABS_ESC/BrakeSysFeatures_0x415/VehYawNonLin_W_Rq ==
  in : Inport
  out : Outport
  wires:
  in/1 -> out/1

== system test_mdl_NI/CAN_Signal/ABS_ESC/BrakeSysFeatures_0x415/Veh_V_ActlBrk ==
  in : Inport
  out : Outport
  wires:
  in/1 -> out/1

== system test_mdl_NI/CAN_Signal/ABS_ESC/BrakeSysFeatures_2_0x416/Abs_B_Falt ==
  in : Inport
  out : Outport
  wires:
  in/1 -> out/1

== system test_mdl_NI/CAN_Signal/ABS_ESC/BrakeSysFeatures_2_0x416/BpedMove_D_Actl ==
  in : Inport
  out : Outport
  wires:
  in/1 -> out/1

== system test_mdl_NI/CAN_Signal/ABS_ESC/BrakeSysFeatures_2_0x416/BpedMove_No_Cnt ==
  in : Inport
  out : Outport
  wires:
  in/1 -> out/1

== system test_mdl_NI/CAN_Signal/ABS_ESC/BrakeSysFeatures_2_0x416/BrkBstrVac_B_Rq ==
  in : Inport
  out : Outport
  wires:
  in/1 -> out/1

== system test_mdl_NI/CAN_Signal/ABS_ESC/BrakeSysFeatures_2_0x416/BrkLamp_B_Rq ==
  in : Inport
  out : Outport
  wires:
  in/1 -> out/1

== system test_mdl_NI/CAN_Signal/ABS_ESC/BrakeSysFeatures_2_0x416/ChimeBrk_B_Rq ==
  in : Inport
  out : Outport
  wires:
  in/1 -> out/1

== system test_mdl_NI/CAN_Signal/ABS_ESC/BrakeSysFeatures_2_0x416/DrvAntiLckLamp_D_Rq ==
  in : Inport
  out : Outport
  wires:
  in/1 -> out/1

== system test_mdl_NI/CAN_Signal/ABS_ESC/BrakeSysFeatures_2_0x416/DrvHdcLampInfo_D_Rq ==
  in : Inport
  out : Outport
  wires:
  in/1 -> out/1

== system test_mdl_NI/CAN_Signal/ABS_ESC/BrakeSysFeatures_2_0x416/DrvHdcMsg_D_Rq ==
  in : Inport
  out : Outport
  wires:
  in/1 -> out/1

== system test_mdl_NI/CAN_Signal/ABS_ESC/BrakeSysFeatures_2_0x416/DrvHdcWarnInfo_D_Rq ==
  in : Inport
  out : Outport
  wires:
  in/1 -> out/1

== system test_mdl_NI/CAN_Signal/ABS_ESC/BrakeSysFeatures_2_0x416/DrvSlipCtlLamp_D_Rq ==
  in : Inport
  out : Outport
  wires:
  in/1 -> out/1

== system test_mdl_NI/CAN_Signal/ABS_ESC/BrakeSysFeatures_2_0x416/DrvSlipCtlMde_D_Ind ==
  in : Inport
  out : Outport
  wires:
  in/1 -> out/1

== system test_mdl_NI/CAN_Signal/ABS_ESC/BrakeSysFeatures_2_0x416/HILL_DESC_MC ==
  in : Inport
  out : Outport
  wires:
  in/1 -> out/1

== system test_mdl_NI/CAN_Signal/ABS_ESC/BrakeSysFeatures_2_0x416/HdcMde_D_Actl ==
  in : Inport
  out : Outport
  wires:
  in/1 -> out/1

== system test_mdl_NI/CAN_Signal/ABS_ESC/BrakeSysFeatures_2_0x416/HsaMde_D_Mem ==
  in : Inport
  out : Outport
  wires:
  in/1 -> out/1

== system test_mdl_NI/CAN_Signal/ABS_ESC/BrakeSysFeatures_2_0x416/RearDiffElckrOpen_B_Rq ==
  in : Inport
  out : Outport
  wires:
  in/1 -> out/1

== system test_mdl_NI/CAN_Signal/ABS_ESC/BrakeSysFeatures_2_0x416/RearDiffLck_Tq2_RqMx ==
  in : Inport
  out : Outport
  wires:
  in/1 -> out/1

== system test_mdl_NI/CAN_Signal/ABS_ESC/BrakeSysFeatures_2_0x416/StabCtlBrk_B_Avail ==
  in : Inport
  out : Outport
  wires:
  in/1 -> out/1

== system test_mdl_NI/CAN_Signal/ABS_ESC/BrakeSysFeatures_2_0x416/TCMode ==
  in : Inport
  out : Outport
  wires:
  in/1 -> out/1

== system test_mdl_NI/CAN_Signal/ABS_ESC/BrakeSysFeatures_2_0x416/TRLR_SWAY_CONFIG_STAT ==
  in : Inport
  out : Outport
  wires:
  in/1 -> out/1

== system test_mdl_NI/CAN_Signal/ABS_ESC/BrakeSysFeatures_2_0x416/TRLR_SWAY_EVNT_IN_PROG ==
  in : Inport
  out : Outport
  wires:
  in/1 -> out/1

== system test_mdl_NI/CAN_Signal/ABS_ESC/BrakeSysFeatures_3_0x41E/ApaBrk_D_Stat ==
  in : Inport
  out : Outport
  wires:
  in/1 -> out/1

== system test_mdl_NI/CAN_Signal/ABS_ESC/BrakeSysFeatures_3_0x41E/AutoHoldMde_D_Ind ==
  in : Inport
  out : Outport
  wires:
  in/1 -> out/1

== system test_mdl_NI/CAN_Signal/ABS_ESC/BrakeSysFeatures_3_0x41E/AutoHoldMsgTxt_D_Rq ==
  in : Inport
  out : Outport
  wires:
  in/1 -> out/1

== system test_mdl_NI/CAN_Signal/ABS_ESC/BrakeSysFeatures_3_0x41E/AutoHoldSwMde_B_Ind ==
  in : Inport
  out : Outport
  wires:
  in/1 -> out/1

== system test_mdl_NI/CAN_Signal/ABS_ESC/BrakeSysFeatures_3_0x41E/BrkBstrVac_D_Stat ==
  in : Inport
  out : Outport
  wires:
  in/1 -> out/1

== system test_mdl_NI/CAN_Signal/ABS_ESC/BrakeSysFeatures_3_0x41E/BrkMdeInhbt_B_RqDsply ==
  in : Inport
  out : Outport
  wires:
  in/1 -> out/1

== system test_mdl_NI/CAN_Signal/ABS_ESC/BrakeSysFeatures_3_0x41E/CtaBrk_D_Stat ==
  in : Inport
  out : Outport
  wires:
  in/1 -> out/1

== system test_mdl_NI/CAN_Signal/ABS_ESC/BrakeSysFeatures_3_0x41E/DrvSlipCtlMdeMsg_D_Rq ==
  in : Inport
  out : Outport
  wires:
  in/1 -> out/1

== system test_mdl_NI/CAN_Signal/ABS_ESC/BrakeSysFeatures_3_0x41E/DrvSlipCtlOffLamp_D_Rq ==
  in : Inport
  out : Outport
  wires:
  in/1 -> out/1

== system test_mdl_NI/CAN_Signal/ABS_ESC/BrakeSysFeatures_3_0x41E/RbaBrk_D_Stat ==
  in : Inport
  out : Outport
  wires:
  in/1 -> out/1

== system test_mdl_NI/CAN_Signal/ABS_ESC/BrakeSysFeatures_3_0x41E/SelDrvMdeAwd_D_Rq ==
  in : Inport
  out : Outport
  wires:
  in/1 -> out/1

== system test_mdl_NI/CAN_Signal/ABS_ESC/BrakeSysFeatures_3_0x41E/SelDrvMdeChassis2_D_Rq ==
  in : Inport
  out : Outport
  wires:
  in/1 -> out/1

== system test_mdl_NI/CAN_Signal/ABS_ESC/BrakeSysFeatures_3_0x41E/SelDrvMdeChassis_D_Rq ==
  in : Inport
  out : Outport
  wires:
  in/1 -> out/1

== system test_mdl_NI/CAN_Signal/ABS_ESC/BrakeSysFeatures_3_0x41E/TrailCtlMsgTxt_D_Rq ==
  in : Inport
  out : Outport
  wires:
  in/1 -> out/1

== system test_mdl_NI/CAN_Signal/ABS_ESC/BrakeSysFeatures_3_0x41E/TrailCtl_D_Stat ==
  in : Inport
  out : Outport
  wires:
  in/1 -> out/1

== system test_mdl_NI/CAN_Signal/ABS_ESC/DesiredTorqBrk_0x213/AbsActv_B_Actl ==
  in : Inport
  out : Outport
  wires:
  in/1 -> out/1

== system test_mdl_NI/CAN_Signal/ABS_ESC/DesiredTorqBrk_0x213/AccBrkActv_B_Actl ==
  in : Inport
  out : Outport
  wires:
  in/1 -> out/1

== system test_mdl_NI/CAN_Signal/ABS_ESC/DesiredTorqBrk_0x213/AccBrkDeny_B_Actl ==
  in : Inport
  out : Outport
  wires:
  in/1 -> out/1

== system test_mdl_NI/CAN_Signal/ABS_ESC/DesiredTorqBrk_0x213/AccBrkDis_B_Actl ==
  in : Inport
  out : Outport
  wires:
  in/1 -> out/1

== system test_mdl_NI/CAN_Signal/ABS_ESC/DesiredTorqBrk_0x213/AccBrkPrchgActv_B_Actl ==
  in : Inport
  out : Outport
  wires:
  in/1 -> out/1

== system test_mdl_NI/CAN_Signal/ABS_ESC/DesiredTorqBrk_0x213/AccBrkTotTqMn_B_Actl ==
  in : Inport
  out : Outport
  wires:
  in/1 -> out/1

== system test_mdl_NI/CAN_Signal/ABS_ESC/DesiredTorqBrk_0x213/AccBrkWarm_B_Actl ==
  in : Inport
  out : Outport
  wires:
  in/1 -> out/1

== system test_mdl_NI/CAN_Signal/ABS_ESC/DesiredTorqBrk_0x213/AccDis_B_ActlEpb ==
  in : Inport
  out : Outport
  wires:
  in/1 -> out/1

== system test_mdl_NI/CAN_Signal/ABS_ESC/DesiredTorqBrk_0x213/AccStopActv_B_ActlBrk ==
  in : Inport
  out : Outport
  wires:
  in/1 -> out/1

== system test_mdl_NI/CAN_Signal/ABS_ESC/DesiredTorqBrk_0x213/CcDis_B_Cmd ==
  in : Inport
  out : Outport
  wires:
  in/1 -> out/1

== system test_mdl_NI/CAN_Signal/ABS_ESC/DesiredTorqBrk_0x213/CmbbBaSensInc_B_Actl ==
  in : Inport
  out : Outport
  wires:
  in/1 -> out/1

== system test_mdl_NI/CAN_Signal/ABS_ESC/DesiredTorqBrk_0x213/CmbbBrkDecel_B_Actl ==
  in : Inport
  out : Outport
  wires:
  in/1 -> out/1

== system test_mdl_NI/CAN_Signal/ABS_ESC/DesiredTorqBrk_0x213/CmbbBrkDis_B_Actl ==
  in : Inport
  out : Outport
  wires:
  in/1 -> out/1

== system test_mdl_NI/CAN_Signal/ABS_ESC/DesiredTorqBrk_0x213/CmbbBrkPrchg_B_Actl ==
  in : Inport
  out : Outport
  wires:
  in/1 -> out/1

== system test_mdl_NI/CAN_Signal/ABS_ESC/DesiredTorqBrk_0x213/CmbbDeny_B_ActlBrk ==
  in : Inport
  out : Outport
  wires:
  in/1 -> out/1

== system test_mdl_NI/CAN_Signal/ABS_ESC/DesiredTorqBrk_0x213/LscmbBrkPrchg_B_Actl ==
  in : Inport
  out : Outport
  wires:
  in/1 -> out/1

== system test_mdl_NI/CAN_Signal/ABS_ESC/DesiredTorqBrk_0x213/LscmbbBaSensInc_B_Actl ==
  in : Inport
  out : Outport
  wires:
  in/1 -> out/1

== system test_mdl_NI/CAN_Signal/ABS_ESC/DesiredTorqBrk_0x213/LscmbbBrkDecel_B_Actl ==
  in : Inport
  out : Outport
  wires:
  in/1 -> out/1

== system test_mdl_NI/CAN_Signal/ABS_ESC/DesiredTorqBrk_0x213/LscmbbBrkDis_B_Actl ==
  in : Inport
  out : Outport
  wires:
  in/1 -> out/1

== system test_mdl_NI/CAN_Signal/ABS_ESC/DesiredTorqBrk_0x213/LscmbbDeny_B_ActlBrk ==
  in : Inport
  out : Outport
  wires:
  in/1 -> out/1

== system test_mdl_NI/CAN_Signal/ABS_ESC/DesiredTorqBrk_0x213/LscmbbMntr_B_Err ==
  in : Inport
  out : Outport
  wires:
  in/1 -> out/1

== system test_mdl_NI/CAN_Signal/ABS_ESC/DesiredTorqBrk_0x213/PrkBrkMsgTxt_D_Rq ==
  in : Inport
  out : Outport
  wires:
  in/1 -> out/1

== system test_mdl_NI/CAN_Signal/ABS_ESC/DesiredTorqBrk_0x213/PrkBrkRedLamp_D_Rq ==
  in : Inport
  out : Outport
  wires:
  in/1 -> out/1

== system test_mdl_NI/CAN_Signal/ABS_ESC/DesiredTorqBrk_0x213/PrkBrkStatus ==
  in : Inport
  out : Outport
  wires:
  in/1 -> out/1

== system test_mdl_NI/CAN_Signal/ABS_ESC/DesiredTorqBrk_0x213/PrkBrkYwLamp_D_Rq ==
  in : Inport
  out : Outport
  wires:
  in/1 -> out/1

== system test_mdl_NI/CAN_Signal/ABS_ESC/DesiredTorqBrk_0x213/PrplDrgCtlActv_B_Actl ==
  in : Inport
  out : Outport
  wires:
  in/1 -> out/1

== system test_mdl_NI/CAN_Signal/ABS_ESC/DesiredTorqBrk_0x213/PrplWhlTot_Tq_RqMx ==
  in : Inport
  out : Outport
  wires:
  in/1 -> out/1

== system test_mdl_NI/CAN_Signal/ABS_ESC/DesiredTorqBrk_0x213/StabCtlBrkActv_B_Actl ==
  in : Inport
  out : Outport
  wires:
  in/1 -> out/1

== system test_mdl_NI/CAN_Signal/ABS_ESC/DesiredTorqBrk_0x213/TracCtlPtActv_B_Actl ==
  in : Inport
  out : Outport
  wires:
  in/1 -> out/1

== system test_mdl_NI/CAN_Signal/ABS_ESC/DesiredTorqBrk_0x213/VehLongOvrGnd_A_Est ==
  in : Inport
  out : Outport
  wires:
  in/1 -> out/1

== system test_mdl_NI/CAN_Signal/ABS_ESC/DesiredTorqBrk_0x213/VehStop_D_Stat ==
  in : Inport
  out : Outport
  wires:
  in/1 -> out/1

== system test_mdl_NI/CAN_Signal/ABS_ESC/DesiredTorqBrk_0x213/VehicleStationary ==
  in : Inport
  out : Outport
  wires:
  in/1 -> out/1

== system test_mdl_NI/CAN_Signal/ABS_ESC/DesiredTorqBrk_2_0x214/PrplWhlRear_Tq_RqMn ==
  in : Inport
  out : Outport
  wires:
  in/1 -> out/1

== system test_mdl_NI/CAN_Signal/ABS_ESC/DesiredTorqBrk_2_0x214/PrplWhlRear_Tq_RqMx ==
  in : Inport
  out : Outport
  wires:
  in/1 -> out/1

== system test_mdl_NI/CAN_Signal/ABS_ESC/DesiredTorqBrk_2_0x214/PrplWhlTot_Tq_RqMn ==
  in : Inport
  out : Outport
  wires:
  in/1 -> out/1

== system test_mdl_NI/CAN_Signal/ABS_ESC/DesiredTorqBrk_2_0x214/PrplWhlTqRqMn_No_Cnt ==
  in : Inport
  out : Outport
  wires:
  in/1 -> out/1

== system test_mdl_NI/CAN_Signal/ABS_ESC/DesiredTorqBrk_2_0x214/PrplWhlTqRqMn_No_Cs ==
  in : Inport
  out : Outport
  wires:
  in/1 -> out/1

== system test_mdl_NI/CAN_Signal/ABS_ESC/DesiredTorqBrk_2_0x214/RgenBrkDynoMde_B_Actl ==
  in : Inport
  out : Outport
  wires:
  in/1 -> out/1

== system test_mdl_NI/CAN_Signal/ABS_ESC/DesiredTorqBrk_2_0x214/RgenTqFalt_B_Actl ==
  in : Inport
  out : Outport
  wires:
  in/1 -> out/1

== system test_mdl_NI/CAN_Signal/ABS_ESC/Global_PATS_SubTarget_0x49/immoSubTarget1Cmd_T1 ==
  in : Inport
  out : Outport
  wires:
  in/1 -> out/1

== system test_mdl_NI/CAN_Signal/ABS_ESC/Global_PATS_SubTarget_0x49/immoSubTarget1Data_T1 ==
  in : Inport
  out : Outport
  wires:
  in/1 -> out/1

== system test_mdl_NI/CAN_Signal/ABS_ESC/SelectDriveModeData2_0x44E/SelDrvMdePos01_D_Stat ==
  in : Inport
  out : Outport
  wires:
  in/1 -> out/1

== system test_mdl_NI/CAN_Signal/ABS_ESC/SelectDriveModeData2_0x44E/SelDrvMdePos02_D_Stat ==
  in : Inport
  out : Outport
  wires:
  in/1 -> out/1

== system test_mdl_NI/CAN_Signal/ABS_ESC/SelectDriveModeData2_0x44E/SelDrvMdePos03_D_Stat ==
  in : Inport
  out : Outport
  wires:
  in/1 -> out/1

== system test_mdl_NI/CAN_Signal/ABS_ESC/SelectDriveModeData2_0x44E/SelDrvMdePos04_D_Stat ==
  in : Inport
  out : Outport
  wires:
  in/1 -> out/1

== system test_mdl_NI/CAN_Signal/ABS_ESC/SelectDriveModeData2_0x44E/SelDrvMdePos05_D_Stat ==
  in : Inport
  out : Outport
  wires:
  in/1 -> out/1

== system test_mdl_NI/CAN_Signal/ABS_ESC/SelectDriveModeData2_0x44E/SelDrvMdePos06_D_Stat ==
  in : Inport
  out : Outport
  wires:
  in/1 -> out/1

== system test_mdl_NI/CAN_Signal/ABS_ESC/SelectDriveModeData2_0x44E/SelDrvMdePos07_D_Stat ==
  in : Inport
  out : Outport
  wires:
  in/1 -> out/1

== system test_mdl_NI/CAN_Signal/ABS_ESC/SelectDriveModeData2_0x44E/SelDrvMdePos08_D_Stat ==
  in : Inport
  out : Outport
  wires:
  in/1 -> out/1

== system test_mdl_NI/CAN_Signal/ABS_ESC/SelectDriveModeData2_0x44E/SelDrvMdePos09_D_Stat ==
  in : Inport
  out : Outport
  wires:
  in/1 -> out/1

== system test_mdl_NI/CAN_Signal/ABS_ESC/SelectDriveModeData2_0x44E/SelDrvMdePos10_D_Stat ==
  in : Inport
  out : Outport
  wires:
  in/1 -> out/1

== system test_mdl_NI/CAN_Signal/ABS_ESC/SelectDriveModeData2_0x44E/SelDrvMdePos11_D_Stat ==
  in : Inport
  out : Outport
  wires:
  in/1 -> out/1

== system test_mdl_NI/CAN_Signal/ABS_ESC/SelectDriveModeData2_0x44E/SelDrvMdePos12_D_Stat ==
  in : Inport
  out : Outport
  wires:
  in/1 -> out/1

== system test_mdl_NI/CAN_Signal/ABS_ESC/SelectDriveModeData_0x420/ActvDrvMde_D2_Stat ==
  in : Inport
  out : Outport
  wires:
  in/1 -> out/1

== system test_mdl_NI/CAN_Signal/ABS_ESC/SelectDriveModeData_0x420/AwdMde_D_RqBrk ==
  in : Inport
  out : Outport
  wires:
  in/1 -> out/1

== system test_mdl_NI/CAN_Signal/ABS_ESC/SelectDriveModeData_0x420/SelDrvMdeMsgTxt_D_Rq ==
  in : Inport
  out : Outport
  wires:
  in/1 -> out/1

== system test_mdl_NI/CAN_Signal/ABS_ESC/SelectDriveModeData_0x420/SelDrvMdePos01_B_Avail ==
  in : Inport
  out : Outport
  wires:
  in/1 -> out/1

== system test_mdl_NI/CAN_Signal/ABS_ESC/SelectDriveModeData_0x420/SelDrvMdePos02_B_Avail ==
  in : Inport
  out : Outport
  wires:
  in/1 -> out/1

== system test_mdl_NI/CAN_Signal/ABS_ESC/SelectDriveModeData_0x420/SelDrvMdePos03_B_Avail ==
  in : Inport
  out : Outport
  wires:
  in/1 -> out/1

== system test_mdl_NI/CAN_Signal/ABS_ESC/SelectDriveModeData_0x420/SelDrvMdePos04_B_Avail ==
  in : Inport
  out : Outport
  wires:
  in/1 -> out/1

== system test_mdl_NI/CAN_Signal/ABS_ESC/SelectDriveModeData_0x420/SelDrvMdePos05_B_Avail ==
  in : Inport
  out : Outport
  wires:
  in/1 -> out/1

== system test_mdl_NI/CAN_Signal/ABS_ESC/SelectDriveModeData_0x420/SelDrvMdePos06_B_Avail ==
  in : Inport
  out : Outport
  wires:
  in/1 -> out/1

== system test_mdl_NI/CAN_Signal/ABS_ESC/SelectDriveModeData_0x420/SelDrvMdePos07_B_Avail ==
  in : Inport
  out : Outport
  wires:
  in/1 -> out/1

== system test_mdl_NI/CAN_Signal/ABS_ESC/SelectDriveModeData_0x420/SelDrvMdePos08_B_Avail ==
  in : Inport
  out : Outport
  wires:
  in/1 -> out/1

== system test_mdl_NI/CAN_Signal/ABS_ESC/SelectDriveModeData_0x420/SelDrvMdePos09_B_Avail ==
  in : Inport
  out : Outport
  wires:
  in/1 -> out/1

== system test_mdl_NI/CAN_Signal/ABS_ESC/SelectDriveModeData_0x420/SelDrvMdePos10_B_Avail ==
  in : Inport
  out : Outport
  wires:
  in/1 -> out/1

== system test_mdl_NI/CAN_Signal/ABS_ESC/SelectDriveModeData_0x420/SelDrvMdePos11_B_Avail ==
  in : Inport
  out : Outport
  wires:
  in/1 -> out/1

== system test_mdl_NI/CAN_Signal/ABS_ESC/SelectDriveModeData_0x420/SelDrvMdePos12_B_Avail ==
  in : Inport
  out : Outport
  wires:
  in/1 -> out/1

== system test_mdl_NI/CAN_Signal/ABS_ESC/SelectDriveModeData_0x420/SelDrvMdePt_D_Rq ==
  in : Inport
  out : Outport
  wires:
  in/1 -> out/1

== system test_mdl_NI/CAN_Signal/ABS_ESC/SelectDriveModeData_0x420/SelDrvMde_D2_Rq ==
  in : Inport
  out : Outport
  wires:
  in/1 -> out/1

== system test_mdl_NI/CAN_Signal/ABS_ESC/SelectDriveModeData_0x420/SelDrvMde_D_Stat ==
  in : Inport
  out : Outport
  wires:
  in/1 -> out/1

== system test_mdl_NI/CAN_Signal/ABS_ESC/SteeringPinion_Data2_0x7F/AwdLatDelta_B_Rq ==
  in : Inport
  out : Outport
  wires:
  in/1 -> out/1

== system test_mdl_NI/CAN_Signal/ABS_ESC/SteeringPinion_Data2_0x7F/AwdLatDelta_Tq_Rq ==
  in : Inport
  out : Outport
  wires:
  in/1 -> out/1

== system test_mdl_NI/CAN_Signal/ABS_ESC/TesterPhysicalResABS_0x768/TesterPhysicalResABS ==
  in : Inport
  out : Outport
  wires:
  in/1 -> out/1

== system test_mdl_NI/CAN_Signal/ABS_ESC/TrailerBrakeData_0x412/TrlrBrk_Pc_Rq ==
  in : Inport
  out : Outport
  wires:
  in/1 -> out/1
